simulink model "PTLo_LosCalc"  (R2016b)
settings: configuration reference "CodeGenConfigSet" (kept outside this file)
values from neighbouring files (symbols this model uses):
  PT_bTrqConv_C = Calibration.Parameter    [init_PTLo_LosCalc.m]
settings Model: Creator=Wollf  LastModifiedBy=Wollf
settings ConfigSetRef: SourceLocation=Base Workspace

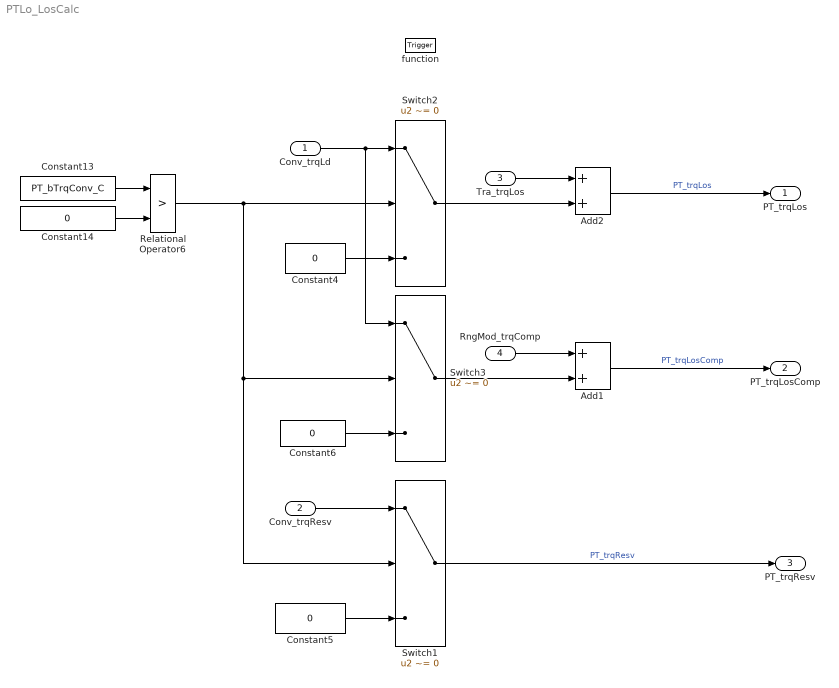
== system PTLo_LosCalc ==
  Conv_trqLd : Inport  Tag=Nm  Description=Application parameter for torque load from the converter  OutMin=-3000  OutMax=3000  OutDataTypeStr=Trq_Nm
  Conv_trqResv : Inport  Tag=Nm  Description=Torque reserve from the converter  Port=2  OutMin=-3000  OutMax=3000  OutDataTypeStr=Trq_Nm
  Tra_trqLos : Inport  Tag=Nm  Description=Gearbox torque loss  Port=3  OutMin=-3000  OutMax=3000  OutDataTypeStr=Trq_Nm
  RngMod_trqComp : Inport  Tag=Nm  Description=torque to be compensated  Port=4  OutMin=-3276.8  OutMax=3276.7  OutDataTypeStr=Trq_Nm
  function : TriggerPort  TriggerType=function-call  VariantControl=Variant
  Add1 : Sum  SaturateOnIntegerOverflow=on  InputSameDT=on
  Add2 : Sum  SaturateOnIntegerOverflow=on  InputSameDT=on
  Constant13 : Constant  Value=PT_bTrqConv_C  OutDataTypeStr=boolean
  Constant14 : Constant  Value=0  OutDataTypeStr=Inherit: Inherit via back propagation
  Constant4 : Constant  Value=0  OutDataTypeStr=Trq_Nm
  Constant5 : Constant  Value=0  OutDataTypeStr=Trq_Nm
  Constant6 : Constant  Value=0  OutDataTypeStr=Trq_Nm
  Relational Operator6 : RelationalOperator  Operator=>  OutDataTypeStr=boolean  RndMeth=Simplest  InputSameDT=on
  Switch1 : Switch  Criteria=u2 ~= 0  SaturateOnIntegerOverflow=on  InputSameDT=on
  Switch2 : Switch  Criteria=u2 ~= 0  SaturateOnIntegerOverflow=on  InputSameDT=on
  Switch3 : Switch  Criteria=u2 ~= 0  SaturateOnIntegerOverflow=on  InputSameDT=on
  PT_trqLos : Outport  Tag=Nm  Description=Parameter for loss torque of the drive train  OutMin=-3000  OutMax=3000  OutDataTypeStr=Trq_Nm
  PT_trqLosComp : Outport  Tag=Nm  Description=Torque loss of the power train  Port=2  OutMin=-3000  OutMax=3000  OutDataTypeStr=Trq_Nm
  PT_trqResv : Outport  Tag=Nm  Description=torque reserve of the drive train  Port=3  OutMin=-3000  OutMax=3000  OutDataTypeStr=Trq_Nm
  wires:
  Constant5/1 -> Switch1/3
  Tra_trqLos/1 -> Add2/1
  Constant14/1 -> Relational Operator6/2
  Switch1/1 -> PT_trqResv/1  "PT_trqResv"
  Add2/1 -> PT_trqLos/1  "PT_trqLos"
  Conv_trqResv/1 -> Switch1/1
  Switch2/1 -> Add2/2
  Constant13/1 -> Relational Operator6/1
  Constant4/1 -> Switch2/3
  Relational Operator6/1 -> Switch2/2, Switch1/2, Switch3/2
  RngMod_trqComp/1 -> Add1/1
  Conv_trqLd/1 -> Switch3/1, Switch2/1
  Add1/1 -> PT_trqLosComp/1  "PT_trqLosComp"
  Switch3/1 -> Add1/2
  Constant6/1 -> Switch3/3
